simulink model "Simulink_PID"  (R2023a)
settings: Solver=VariableStepAuto  StartTime=0.0  StopTime=30  RelTol=1e-3
undefined symbols (not defined in the file): DiscIntNeverNeededParam
libraries: simulink x2
settings Model: Creator=usuario  LastModifiedBy=rodri

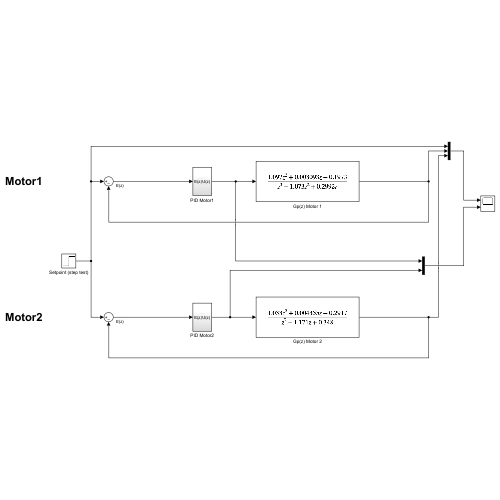
[thumbnail: Simulink's stored preview of the top-level diagram]
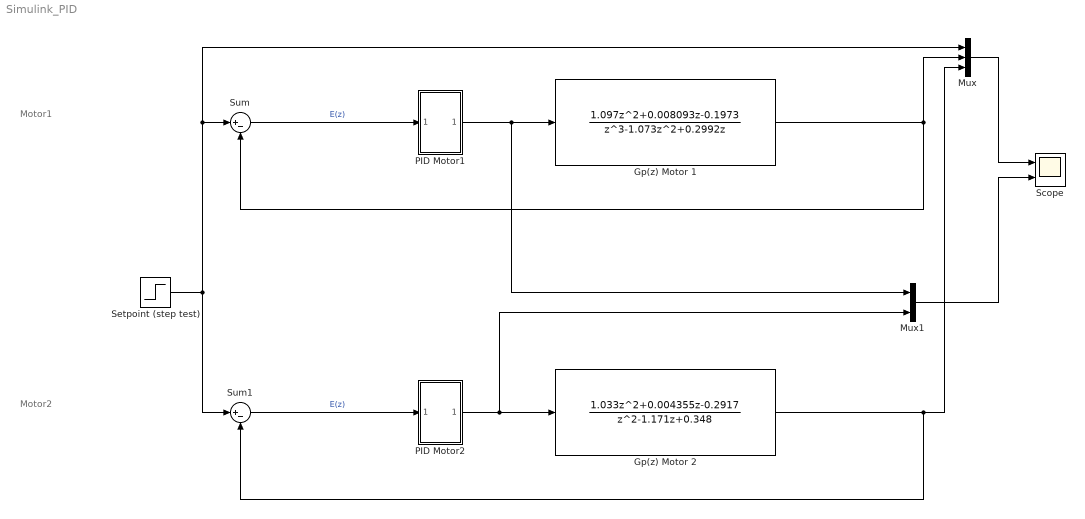
== system Simulink_PID ==
  note: Motor1
  note: Motor2
  Gp(z) Motor 1 : DiscreteTransferFcn  Numerator=[1.097 0.008093 -0.1973]  Denominator=[1 -1.073 0.2992 0]
  Gp(z) Motor 2 : DiscreteTransferFcn  Numerator=[1.033 0.004355 -0.2917]  Denominator=[1 -1.171 0.348]
  Mux : Mux  Inputs=3
  Mux1 : Mux  Inputs=2
  PID Motor1 : Subsystem
  PID Motor2 : Subsystem
  Scope : Scope  NumInputPorts=2
  Setpoint (step test) : Step  After=5  SampleTime=1
  Sum : Sum  Inputs=|+-
  Sum1 : Sum  Inputs=|+-
  wires:
  Setpoint (step test)/1 -> Mux/1, Sum/1, Sum1/1
  Mux/1 -> Scope/1
  PID Motor1/1(U(z)) -> Mux1/1, Gp(z) Motor 1/1
  Sum/1 -> PID Motor1/1(E(z))  "E(z)"
  Gp(z) Motor 1/1 -> Sum/2, Mux/2
  Gp(z) Motor 2/1 -> Sum1/2, Mux/3
  PID Motor2/1(U(z)) -> Mux1/2, Gp(z) Motor 2/1
  Sum1/1 -> PID Motor2/1(E(z))  "E(z)"
  Mux1/1 -> Scope/2

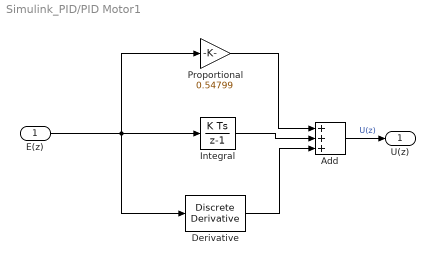
== system Simulink_PID/PID Motor1 ==
  E(z) : Inport
  Add : Sum  Inputs=+++
  Derivative : simulink/Discrete/Discrete Derivative  gainval=0.182223  ICPrevScaledInput=0.0  OutMin=[]  OutMax=[]  OutDataType=fixdt(1, 16)  OutScaling=2^-10  DoSatur=off
  Integral : DiscreteIntegrator  gainval=0.22643  SampleTime=-1  ICPrevOutput=DiscIntNeverNeededParam  ICPrevScaledInput=DiscIntNeverNeededParam
  Proportional : Gain  Gain=0.54799
  U(z) : Outport
  wires:
  Derivative/1 -> Add/3
  Proportional/1 -> Add/1
  Integral/1 -> Add/2
  Add/1 -> U(z)/1  "U(z)"
  E(z)/1 -> Derivative/1, Proportional/1, Integral/1

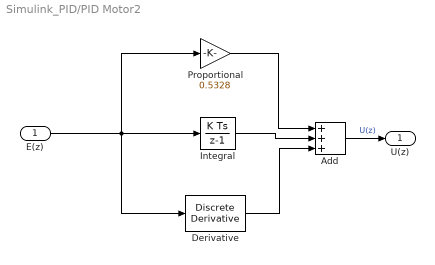
== system Simulink_PID/PID Motor2 ==
  E(z) : Inport
  Add : Sum  Inputs=+++
  Derivative : simulink/Discrete/Discrete Derivative  gainval=0.1868  ICPrevScaledInput=0.0  OutMin=[]  OutMax=[]  OutDataType=fixdt(1, 16)  OutScaling=2^-10  DoSatur=off
  Integral : DiscreteIntegrator  gainval=0.2022  SampleTime=-1  ICPrevOutput=DiscIntNeverNeededParam  ICPrevScaledInput=DiscIntNeverNeededParam
  Proportional : Gain  Gain=0.5328
  U(z) : Outport
  wires:
  Derivative/1 -> Add/3
  Proportional/1 -> Add/1
  Integral/1 -> Add/2
  Add/1 -> U(z)/1  "U(z)"
  E(z)/1 -> Derivative/1, Proportional/1, Integral/1
